simulink model "EndSoc"  (R2021b)
settings: Solver=FixedStepAuto  StartTime=0.0  StopTime=500  FixedStep=0.001  RelTol=1e-3
undefined symbols (not defined in the file): CtrlSampleTime, DiscIntNeverNeededParam
settings Model: Creator=miche  LastModifiedBy=miche

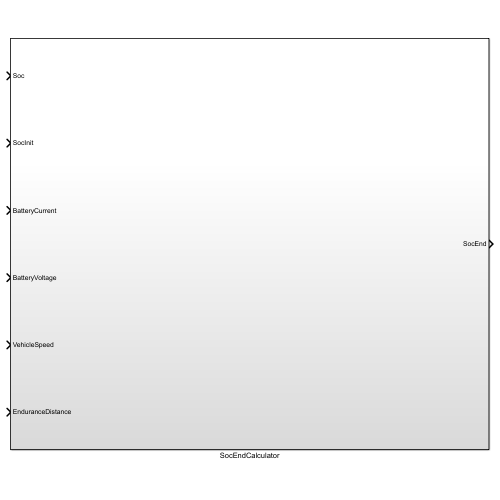
[thumbnail: Simulink's stored preview of the top-level diagram]
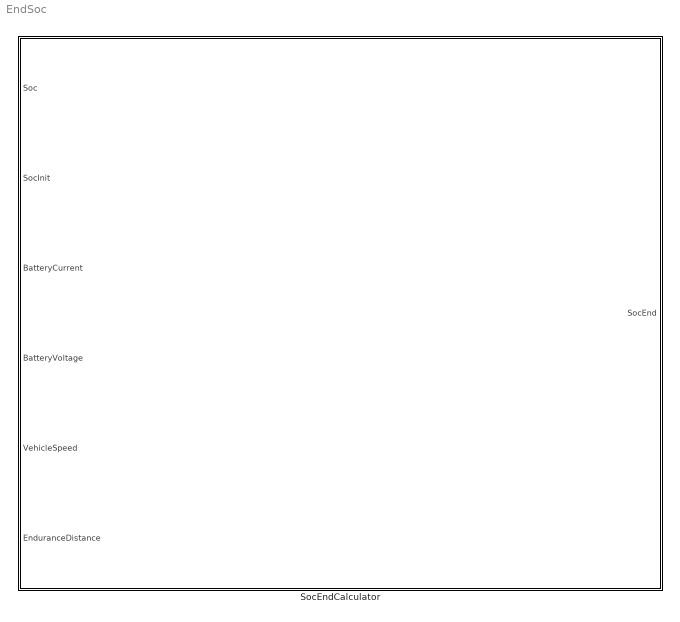
== system EndSoc ==
  SocEndCalculator : Subsystem

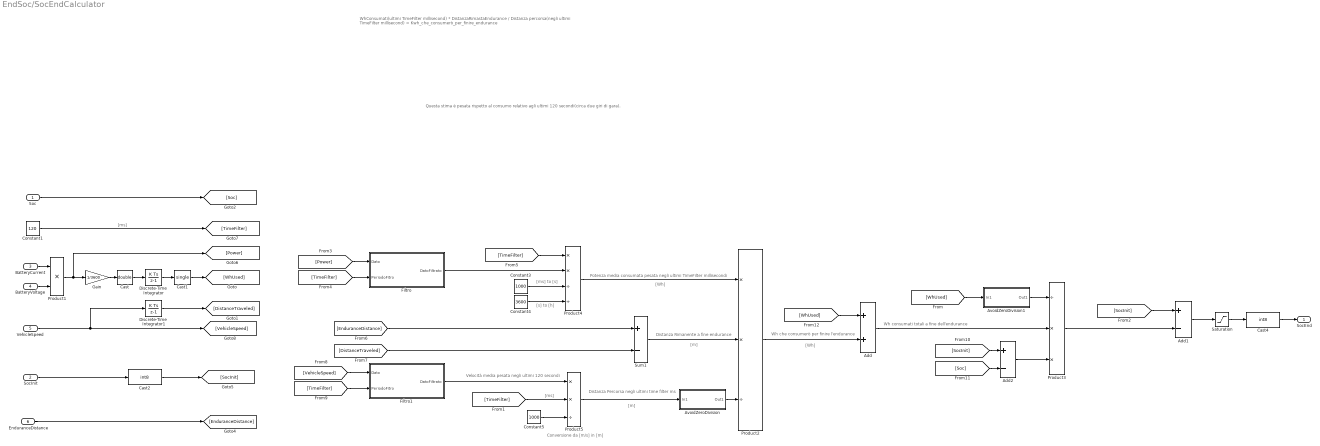
== system EndSoc/SocEndCalculator ==
  note: [ms]
  note: [Wh]
  note: [s] to [h]
  note: [Wh]
  note: [m]
  note: [m]
  note: Distanza Rimanente a fine endurance
  note: Wh consumati totali a fine dell'endurance
  note: Distanza Percorsa negli ultimi time filter ms
  note: [ms]
  note: Velocità media pesata negli ultimi 120 secondi
  note: Potenza media consumata pesata negli ultimi TimeFilter millisecondi
  note: Questa stima è pesata rispetto al consumo relativo agli ultimi 120 secondi(circa due giri di gara).
  note: WhConsumati(ultimi TimeFilter millisecond) * DistanzaRimastaEndurance / Distanza percorsa(negli ultimi TimeFilter millisecond) = Kwh_che_consumerò_per_finire_endurance
  note: Conversione da [m/s] in [m]
  note: [ms] to [s]
  note: Wh che consumerò per finire l'endurance
  Soc : Inport
  SocInit : Inport  Port=2
  BatteryCurrent : Inport  Port=3
  BatteryVoltage : Inport  Port=4
  VehicleSpeed : Inport  Port=5  OutDataTypeStr=single
  EnduranceDistance : Inport  Port=6  OutDataTypeStr=uint32
  Add : Sum
  Add1 : Sum  Inputs=+-
  Add2 : Sum  Inputs=+-
  AvoidZeroDivision : Subsystem
  AvoidZeroDivision1 : Subsystem
  Cast : DataTypeConversion  OutDataTypeStr=double
  Cast1 : DataTypeConversion  OutDataTypeStr=single
  Cast2 : DataTypeConversion  OutDataTypeStr=int8
  Cast4 : DataTypeConversion  OutDataTypeStr=int8
  Constant1 : Constant  Value=120
  Constant3 : Constant  Value=1000  OutDataTypeStr=single
  Constant4 : Constant  Value=3600  OutDataTypeStr=single
  Constant5 : Constant  Value=1000  OutDataTypeStr=single
  Discrete-Time Integrator : DiscreteIntegrator  SampleTime=-1  ICPrevOutput=DiscIntNeverNeededParam  ICPrevScaledInput=DiscIntNeverNeededParam
  Discrete-Time Integrator1 : DiscreteIntegrator  SampleTime=-1  ICPrevOutput=DiscIntNeverNeededParam  ICPrevScaledInput=DiscIntNeverNeededParam
  Filtro : Subsystem
  Filtro1 : Subsystem
  Gain : Gain  Gain=1/3600
  Product1 : Product
  Product2 : Product  Inputs=**/
  Product3 : Product  Inputs=/**
  Product4 : Product  Inputs=**//
  Product5 : Product  Inputs=**/
  Saturation : Saturate  UpperLimit=127  LowerLimit=-127
  Sum1 : Sum  Inputs=+-
  SocEnd : Outport  OutDataTypeStr=int8
  wires:
  Product1/1 -> [Power], Gain/1
  SocInit/1 -> Cast2/1
  EnduranceDistance/1 -> [EnduranceDistance]
  BatteryCurrent/1 -> Product1/1
  BatteryVoltage/1 -> Product1/2
  Discrete-Time Integrator/1 -> Cast1/1
  Gain/1 -> Cast/1
  Cast/1 -> Discrete-Time Integrator/1
  Discrete-Time Integrator1/1 -> [DistanceTraveled]
  VehicleSpeed/1 -> Discrete-Time Integrator1/1, [VehicleSpeed]
  [Power] -> Filtro/1(Dato)
  Constant1/1 -> [TimeFilter]
  [TimeFilter] -> Filtro/2(PeriodoFitro)
  [TimeFilter] -> Product4/1
  Constant3/1 -> Product4/3
  Constant4/1 -> Product4/4
  Product4/1 -> Product2/1
  [EnduranceDistance] -> Sum1/1
  [DistanceTraveled] -> Sum1/2
  Sum1/1 -> Product2/2
  [VehicleSpeed] -> Filtro1/1(Dato)
  [TimeFilter] -> Filtro1/2(PeriodoFitro)
  Constant5/1 -> Product5/3
  [TimeFilter] -> Product5/2
  Filtro1/1(DatoFiltrato) -> Product5/1
  Product5/1 -> AvoidZeroDivision/1(In1)
  AvoidZeroDivision/1(Out1) -> Product2/3
  Soc/1 -> [Soc]
  Saturation/1 -> Cast4/1
  Cast4/1 -> SocEnd/1
  Product2/1 -> Add/2
  Add/1 -> Product3/2
  [WhUsed] -> AvoidZeroDivision1/1(In1)
  AvoidZeroDivision1/1(Out1) -> Product3/1
  Product3/1 -> Add1/2
  [SocInit] -> Add1/1
  Cast2/1 -> [SocInit]
  Add1/1 -> Saturation/1
  [SocInit] -> Add2/1
  [Soc] -> Add2/2
  Add2/1 -> Product3/3
  [WhUsed] -> Add/1
  Filtro/1(DatoFiltrato) -> Product4/2
  Cast1/1 -> [WhUsed]

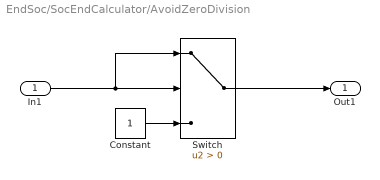
== system EndSoc/SocEndCalculator/AvoidZeroDivision ==
  In1 : Inport
  Constant : Constant  OutDataTypeStr=single
  Switch : Switch  Criteria=u2 > Threshold
  Out1 : Outport
  wires:
  In1/1 -> Switch/1, Switch/2
  Switch/1 -> Out1/1
  Constant/1 -> Switch/3

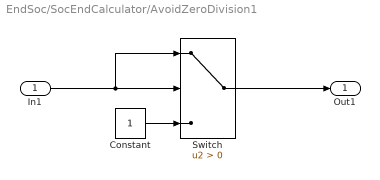
== system EndSoc/SocEndCalculator/AvoidZeroDivision1 ==
  In1 : Inport
  Constant : Constant  OutDataTypeStr=single
  Switch : Switch  Criteria=u2 > Threshold
  Out1 : Outport
  wires:
  Constant/1 -> Switch/3
  Switch/1 -> Out1/1
  In1/1 -> Switch/2, Switch/1

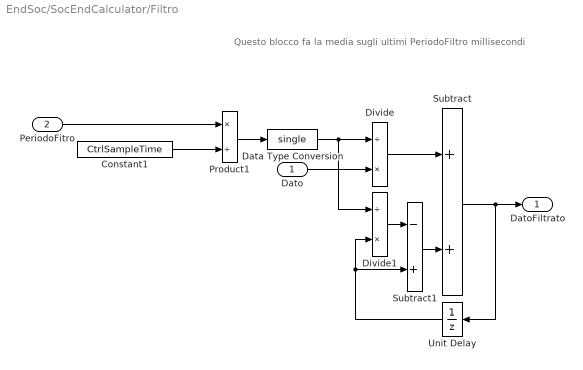
== system EndSoc/SocEndCalculator/Filtro ==
  note: Questo blocco fa la media sugli ultimi PeriodoFiltro millisecondi
  Dato : Inport  OutDataTypeStr=single
  PeriodoFitro : Inport  Port=2  OutDataTypeStr=uint32
  Constant1 : Constant  Value=CtrlSampleTime  OutDataTypeStr=uint32
  Data Type Conversion : DataTypeConversion  OutDataTypeStr=single
  Divide : Product  Inputs=/*  OutDataTypeStr=single
  Divide1 : Product  Inputs=/*  OutDataTypeStr=single
  Product1 : Product  Inputs=*/  OutDataTypeStr=uint32
  Subtract : Sum  OutDataTypeStr=single
  Subtract1 : Sum  Inputs=-+  OutDataTypeStr=single
  Unit Delay : UnitDelay  SampleTime=-1  HasFrameUpgradeWarning=on
  DatoFiltrato : Outport  OutDataTypeStr=single  VectorParamsAs1DForOutWhenUnconnected=off
  wires:
  Data Type Conversion/1 -> Divide/1, Divide1/1
  PeriodoFitro/1 -> Product1/1
  Dato/1 -> Divide/2
  Subtract/1 -> Unit Delay/1, DatoFiltrato/1
  Divide/1 -> Subtract/1
  Divide1/1 -> Subtract1/1
  Subtract1/1 -> Subtract/2
  Product1/1 -> Data Type Conversion/1
  Unit Delay/1 -> Divide1/2, Subtract1/2
  Constant1/1 -> Product1/2

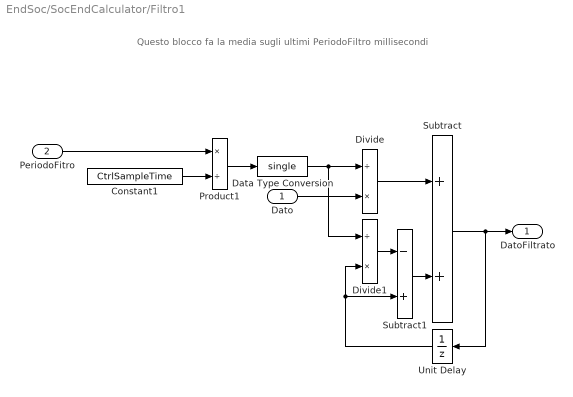
== system EndSoc/SocEndCalculator/Filtro1 ==
  note: Questo blocco fa la media sugli ultimi PeriodoFiltro millisecondi
  Dato : Inport  OutDataTypeStr=single
  PeriodoFitro : Inport  Port=2  OutDataTypeStr=uint32
  Constant1 : Constant  Value=CtrlSampleTime  OutDataTypeStr=uint32
  Data Type Conversion : DataTypeConversion  OutDataTypeStr=single
  Divide : Product  Inputs=/*  OutDataTypeStr=single
  Divide1 : Product  Inputs=/*  OutDataTypeStr=single
  Product1 : Product  Inputs=*/  OutDataTypeStr=uint32
  Subtract : Sum  OutDataTypeStr=single
  Subtract1 : Sum  Inputs=-+  OutDataTypeStr=single
  Unit Delay : UnitDelay  SampleTime=-1  HasFrameUpgradeWarning=on
  DatoFiltrato : Outport  OutDataTypeStr=single  VectorParamsAs1DForOutWhenUnconnected=off
  wires:
  Unit Delay/1 -> Subtract1/2, Divide1/2
  Product1/1 -> Data Type Conversion/1
  Subtract1/1 -> Subtract/2
  Divide1/1 -> Subtract1/1
  Divide/1 -> Subtract/1
  Subtract/1 -> DatoFiltrato/1, Unit Delay/1
  Dato/1 -> Divide/2
  PeriodoFitro/1 -> Product1/1
  Data Type Conversion/1 -> Divide1/1, Divide/1
  Constant1/1 -> Product1/2
